simulink model "PubIfDecisionTOS_MDL"  (R2020b)
settings: configuration reference "DspaceConfig" (kept outside this file)
PostLoadFcn:
  | if any(exist('dsrtsu_mdlpostloadfcn', 'file') ~= 0), dsrtsu_mdlpostloadfcn('Execute', bdroot); end
InitFcn:
  | , if any(exist('dsmpb_private', 'file') ~= 0), dsmpb_private('dsmpb_mdlclblib', 'Init', bdroot); end,
undefined symbols (not defined in the file or in its folder): C_TOS_ACCEgoRAxletoFbumplength_m, C_TOS_ACCTargetFront_Flag, C_TOS_AEBJAPedObjDxThre_Val, C_TOS_AEBJAPedObjDyThre_Val, C_TOS_AEBJATargetSize_Val, C_TOS_AEBJAVehObjDxThre_Val, C_TOS_AEBJAVehObjDyThre_Val, C_TOS_AEBJuncPedTargetSize_Val, C_TOS_AEBLatObjDxThre_Val, C_TOS_AEBLatPedDyThre_Val, C_TOS_AEBLatTargetSize_Val, C_TOS_AEBLongTargetInEgoFront_Flag, C_TOS_axAbsGround_Parameter, C_TOS_CameraConfirmedFlag, C_TOS_CNsubjWidth, C_TOS_CurrentLaneCoreMinWidth_Val, C_TOS_CutInProb_Val_Zero, C_TOS_CutOutProb_Val_Zero, C_TOS_D2R_Val, C_TOS_DefaultValueObjectToCenterLine_dy, C_TOS_EgoCarWidth_Val, C_TOS_EgoDxRefPoint_m, C_TOS_EgoRAxletoFbumplength_m, C_TOS_HalfWidthVehicle_Con, C_TOS_HWA_CurrentLaneFlag, C_TOS_HWA_LeftLaneFlag, C_TOS_HWA_MovingDir_Vaild, C_TOS_HWA_MovState_Vaild, C_TOS_HWA_RightLaneFlag, C_TOS_LaneLineCourseErrorFront, C_TOS_LaneLineCourseErrorRear, C_TOS_MotorbikeDefaultWidth_m, C_TOS_NumberOfEffectiveTargets, C_TOS_Obj_Age_Val, C_TOS_Objdx_Constraint_Val, C_TOS_ObjectDefaultWidth_m, C_TOS_ObjInCurrentLane_Val, C_TOS_ObjInCurrentLaneValid, C_TOS_ObjInLeftLaneValid, C_TOS_ObjInRightLaneValid, C_TOS_ObjNotInCurrentLane_Val, C_TOS_ObjNotREElementType, C_TOS_ObjPredictDis_dy_ConstantVal_Zeros, C_TOS_ObjToCenterLine_ConstantVal_Zeros, C_TOS_OFMObjIDInvilad_Val, C_TOS_PIL_LatDisCons_Val_zero, C_TOS_PIL_ObjectCutInFlag_b, C_TOS_PIL_ObjectCutOutFlag_b, C_TOS_PIL_ObjLaneProb_al_Val, C_TOS_PP_ObjFusType_FC_Confirm_b, C_TOS_PP_ObjFusType_FC_FR_Confirm_b, C_TOS_PP_ObjFusType_FR_Confirm_b, C_TOS_RE_80BoolDefault_Val, C_TOS_RE_80Single181Default_Val, C_TOS_RE_80Single255Default_Val, C_TOS_RE_80Uint8Default_Val, C_TOS_RE_D2R, C_TOS_RE_D_180_Val, C_TOS_RE_InvalidObjectID_Val, C_TOS_RE_InvalidTargetChainDir_Val ... (+142)
libraries: simulink x1650, TOS_LIB x361, canfdmsglib x14
(part 59 of 69)

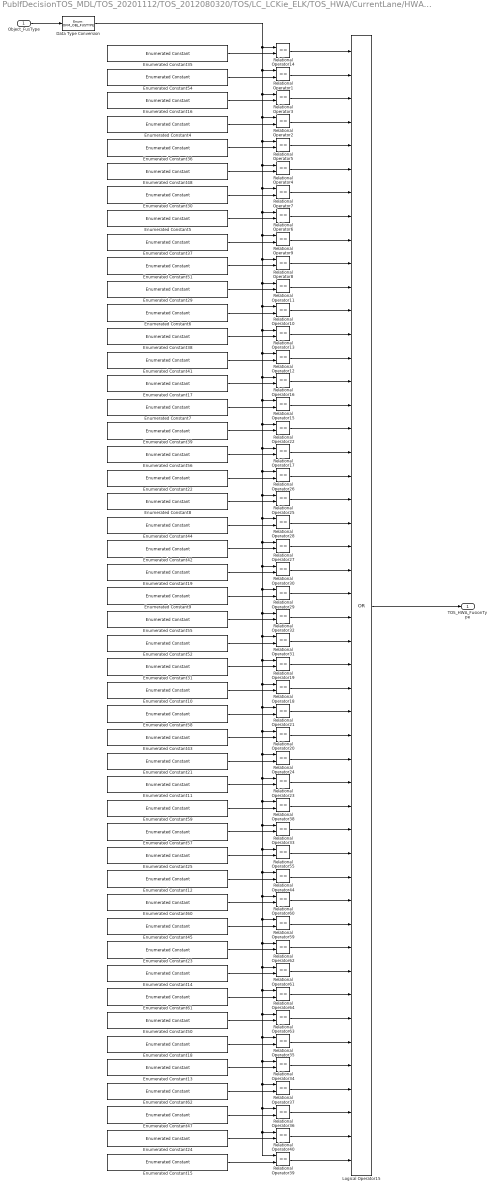
== system PubIfDecisionTOS_MDL/TOS_20201112/TOS_2012080320/TOS/LC_LCKie_ELK/TOS_HWA/CurrentLane/HWA_CurrentLane_Target/HWA_CLF_Target_3/HWA_CLR_Target/HWA_CLR_Target/HWA_CurrentRear_FusionType/FusionType ==
  Object_FusType : Inport
  Data Type Conversion : DataTypeConversion  OutDataTypeStr=Enum: OFM_OBJ_FUSTYPE
  Enumerated Constant10 : simulink/Sources/Enumerated Constant  OutDataTypeStr=Enum: OFM_OBJ_FUSTYPE  Value=OFM_OBJ_FUSTYPE.FC_FR_CR_BR  SampleTime=inf
      settings: AttributesFormatString=OFM_OBJ_FUSTYPE.FC_FR_CR_BR=43
  Enumerated Constant11 : simulink/Sources/Enumerated Constant  OutDataTypeStr=Enum: OFM_OBJ_FUSTYPE  Value=OFM_OBJ_FUSTYPE.FC_FR_CL_CR_BR  SampleTime=inf
      settings: AttributesFormatString=OFM_OBJ_FUSTYPE.FC_FR_CL_CR_BR=47
  Enumerated Constant12 : simulink/Sources/Enumerated Constant  OutDataTypeStr=Enum: OFM_OBJ_FUSTYPE  Value=OFM_OBJ_FUSTYPE.FC_FR_BL_BR  SampleTime=inf
      settings: AttributesFormatString=OFM_OBJ_FUSTYPE.FC_FR_BL_BR=51
  Enumerated Constant13 : simulink/Sources/Enumerated Constant  OutDataTypeStr=Enum: OFM_OBJ_FUSTYPE  Value=OFM_OBJ_FUSTYPE.FC_FR_CR_BL_BR  SampleTime=inf
      settings: AttributesFormatString=OFM_OBJ_FUSTYPE.FC_FR_CR_BL_BR=59
  Enumerated Constant14 : simulink/Sources/Enumerated Constant  OutDataTypeStr=Enum: OFM_OBJ_FUSTYPE  Value=OFM_OBJ_FUSTYPE.FC_FR_CL_BL_BR  SampleTime=inf
      settings: AttributesFormatString=OFM_OBJ_FUSTYPE.FC_FR_CL_BL_BR=55
  Enumerated Constant15 : simulink/Sources/Enumerated Constant  OutDataTypeStr=Enum: OFM_OBJ_FUSTYPE  Value=OFM_OBJ_FUSTYPE.FC_FR_CL_CR_BL_BR  SampleTime=inf
      settings: AttributesFormatString=OFM_OBJ_FUSTYPE.FC_FR_CL_CR_BL_BR=63
  Enumerated Constant16 : simulink/Sources/Enumerated Constant  OutDataTypeStr=Enum: OFM_OBJ_FUSTYPE  Value=OFM_OBJ_FUSTYPE.FR_BL  SampleTime=inf
      settings: AttributesFormatString=OFM_OBJ_FUSTYPE.FR_BL = 18
  Enumerated Constant17 : simulink/Sources/Enumerated Constant  OutDataTypeStr=Enum: OFM_OBJ_FUSTYPE  Value=OFM_OBJ_FUSTYPE.FR_CL_CR_BL  SampleTime=inf
      settings: AttributesFormatString=OFM_OBJ_FUSTYPE.FR_CL_CR_BL = 30
  Enumerated Constant18 : simulink/Sources/Enumerated Constant  OutDataTypeStr=Enum: OFM_OBJ_FUSTYPE  Value=OFM_OBJ_FUSTYPE.FR_CR_BL_BR  SampleTime=inf
      settings: AttributesFormatString=OFM_OBJ_FUSTYPE.FR_CR_BL_BR = 58
  Enumerated Constant19 : simulink/Sources/Enumerated Constant  OutDataTypeStr=Enum: OFM_OBJ_FUSTYPE  Value=OFM_OBJ_FUSTYPE.FR_CL_BR  SampleTime=inf
      settings: AttributesFormatString=OFM_OBJ_FUSTYPE.FR_CL_BR = 38
  Enumerated Constant21 : simulink/Sources/Enumerated Constant  OutDataTypeStr=Enum: OFM_OBJ_FUSTYPE  Value=OFM_OBJ_FUSTYPE.FR_CL_CR_BR  SampleTime=inf
      settings: AttributesFormatString=OFM_OBJ_FUSTYPE.FR_CL_CR_BR = 46
  Enumerated Constant22 : simulink/Sources/Enumerated Constant  OutDataTypeStr=Enum: OFM_OBJ_FUSTYPE  Value=OFM_OBJ_FUSTYPE.FR_BR  SampleTime=inf
      settings: AttributesFormatString=OFM_OBJ_FUSTYPE.FR_BR = 34
  Enumerated Constant23 : simulink/Sources/Enumerated Constant  OutDataTypeStr=Enum: OFM_OBJ_FUSTYPE  Value=OFM_OBJ_FUSTYPE.FR_CL_BL_BR  SampleTime=inf
      settings: AttributesFormatString=OFM_OBJ_FUSTYPE.FR_CL_BL_BR = 54
  Enumerated Constant24 : simulink/Sources/Enumerated Constant  OutDataTypeStr=Enum: OFM_OBJ_FUSTYPE  Value=OFM_OBJ_FUSTYPE.FR_CL_CR_BL_BR  SampleTime=inf
      settings: AttributesFormatString=OFM_OBJ_FUSTYPE.FR_CL_CR_BL_BR = 62
  Enumerated Constant25 : simulink/Sources/Enumerated Constant  OutDataTypeStr=Enum: OFM_OBJ_FUSTYPE  Value=OFM_OBJ_FUSTYPE.FR_BL_BR  SampleTime=inf
      settings: AttributesFormatString=OFM_OBJ_FUSTYPE.FR_BL_BR = 50
  Enumerated Constant29 : simulink/Sources/Enumerated Constant  OutDataTypeStr=Enum: OFM_OBJ_FUSTYPE  Value=OFM_OBJ_FUSTYPE.FR_CR_BL  SampleTime=inf
      settings: AttributesFormatString=OFM_OBJ_FUSTYPE.FR_CR_BL = 26
  Enumerated Constant30 : simulink/Sources/Enumerated Constant  OutDataTypeStr=Enum: OFM_OBJ_FUSTYPE  Value=OFM_OBJ_FUSTYPE.FR_CL_BL  SampleTime=inf
      settings: AttributesFormatString=OFM_OBJ_FUSTYPE.FR_CL_BL = 22
  Enumerated Constant31 : simulink/Sources/Enumerated Constant  OutDataTypeStr=Enum: OFM_OBJ_FUSTYPE  Value=OFM_OBJ_FUSTYPE.FR_CR_BR  SampleTime=inf
      settings: AttributesFormatString=OFM_OBJ_FUSTYPE.FR_CR_BR = 42
  Enumerated Constant35 : simulink/Sources/Enumerated Constant  OutDataTypeStr=Enum: OFM_OBJ_FUSTYPE  Value=OFM_OBJ_FUSTYPE.BL  SampleTime=inf
      settings: AttributesFormatString=OFM_OBJ_FUSTYPE.BL = 16
  Enumerated Constant36 : simulink/Sources/Enumerated Constant  OutDataTypeStr=Enum: OFM_OBJ_FUSTYPE  Value=OFM_OBJ_FUSTYPE.CL_BL  SampleTime=inf
      settings: AttributesFormatString=OFM_OBJ_FUSTYPE.CL_BL=20
  Enumerated Constant37 : simulink/Sources/Enumerated Constant  OutDataTypeStr=Enum: OFM_OBJ_FUSTYPE  Value=OFM_OBJ_FUSTYPE.CR_BL  SampleTime=inf
      settings: AttributesFormatString=OFM_OBJ_FUSTYPE.CR_BL = 24
  Enumerated Constant38 : simulink/Sources/Enumerated Constant  OutDataTypeStr=Enum: OFM_OBJ_FUSTYPE  Value=OFM_OBJ_FUSTYPE.CL_CR_BL  SampleTime=inf
      settings: AttributesFormatString=OFM_OBJ_FUSTYPE.CL_CR_BL=28
  Enumerated Constant39 : simulink/Sources/Enumerated Constant  OutDataTypeStr=Enum: OFM_OBJ_FUSTYPE  Value=OFM_OBJ_FUSTYPE.BR  SampleTime=inf
      settings: AttributesFormatString=OFM_OBJ_FUSTYPE.BR = 32
  Enumerated Constant4 : simulink/Sources/Enumerated Constant  OutDataTypeStr=Enum: OFM_OBJ_FUSTYPE  Value=OFM_OBJ_FUSTYPE.FC_FR_BL  SampleTime=inf
      settings: AttributesFormatString=OFM_OBJ_FUSTYPE.FC_FR_BL=19
  Enumerated Constant41 : simulink/Sources/Enumerated Constant  OutDataTypeStr=Enum: OFM_OBJ_FUSTYPE  Value=OFM_OBJ_FUSTYPE.FC_CL_CR_BL  SampleTime=inf
      settings: AttributesFormatString=OFM_OBJ_FUSTYPE.FC_CL_CR_BL = 29
  Enumerated Constant42 : simulink/Sources/Enumerated Constant  OutDataTypeStr=Enum: OFM_OBJ_FUSTYPE  Value=OFM_OBJ_FUSTYPE.FC_CL_BR  SampleTime=inf
      settings: AttributesFormatString=OFM_OBJ_FUSTYPE.FC_CL_BR = 37
  Enumerated Constant43 : simulink/Sources/Enumerated Constant  OutDataTypeStr=Enum: OFM_OBJ_FUSTYPE  Value=OFM_OBJ_FUSTYPE.FC_CL_CR_BR  SampleTime=inf
      settings: AttributesFormatString=OFM_OBJ_FUSTYPE.FC_CL_CR_BR = 45
  Enumerated Constant44 : simulink/Sources/Enumerated Constant  OutDataTypeStr=Enum: OFM_OBJ_FUSTYPE  Value=OFM_OBJ_FUSTYPE.CL_BR  SampleTime=inf
      settings: AttributesFormatString=OFM_OBJ_FUSTYPE.CL_BR = 36
  Enumerated Constant45 : simulink/Sources/Enumerated Constant  OutDataTypeStr=Enum: OFM_OBJ_FUSTYPE  Value=OFM_OBJ_FUSTYPE.FC_CL_BL_BR  SampleTime=inf
      settings: AttributesFormatString=OFM_OBJ_FUSTYPE.FC_CL_BL_BR = 53
  Enumerated Constant47 : simulink/Sources/Enumerated Constant  OutDataTypeStr=Enum: OFM_OBJ_FUSTYPE  Value=OFM_OBJ_FUSTYPE.FC_CL_CR_BL_BR  SampleTime=inf
      settings: AttributesFormatString=OFM_OBJ_FUSTYPE.FC_CL_CR_BL_BR = 61
  Enumerated Constant48 : simulink/Sources/Enumerated Constant  OutDataTypeStr=Enum: OFM_OBJ_FUSTYPE  Value=OFM_OBJ_FUSTYPE.FC_CL_BL  SampleTime=inf
      settings: AttributesFormatString=OFM_OBJ_FUSTYPE.FC_CL_BL = 21
  Enumerated Constant5 : simulink/Sources/Enumerated Constant  OutDataTypeStr=Enum: OFM_OBJ_FUSTYPE  Value=OFM_OBJ_FUSTYPE.FC_FR_CL_BL  SampleTime=inf
      settings: AttributesFormatString=OFM_OBJ_FUSTYPE.FC_FR_CL_BL=23
  Enumerated Constant50 : simulink/Sources/Enumerated Constant  OutDataTypeStr=Enum: OFM_OBJ_FUSTYPE  Value=OFM_OBJ_FUSTYPE.FC_CR_BL_BR  SampleTime=inf
      settings: AttributesFormatString=OFM_OBJ_FUSTYPE.FC_CR_BL_BR = 57
  Enumerated Constant51 : simulink/Sources/Enumerated Constant  OutDataTypeStr=Enum: OFM_OBJ_FUSTYPE  Value=OFM_OBJ_FUSTYPE.FC_CR_BL  SampleTime=inf
      settings: AttributesFormatString=OFM_OBJ_FUSTYPE.FC_CR_BL = 25
  Enumerated Constant52 : simulink/Sources/Enumerated Constant  OutDataTypeStr=Enum: OFM_OBJ_FUSTYPE  Value=OFM_OBJ_FUSTYPE.FC_CR_BR  SampleTime=inf
      settings: AttributesFormatString=OFM_OBJ_FUSTYPE.FC_CR_BR = 41
  Enumerated Constant54 : simulink/Sources/Enumerated Constant  OutDataTypeStr=Enum: OFM_OBJ_FUSTYPE  Value=OFM_OBJ_FUSTYPE.FC_BL  SampleTime=inf
      settings: AttributesFormatString=OFM_OBJ_FUSTYPE.FC_BL = 17
  Enumerated Constant55 : simulink/Sources/Enumerated Constant  OutDataTypeStr=Enum: OFM_OBJ_FUSTYPE  Value=OFM_OBJ_FUSTYPE.CR_BR  SampleTime=inf
      settings: AttributesFormatString=OFM_OBJ_FUSTYPE.CR_BR = 40
  Enumerated Constant56 : simulink/Sources/Enumerated Constant  OutDataTypeStr=Enum: OFM_OBJ_FUSTYPE  Value=OFM_OBJ_FUSTYPE.FC_BR  SampleTime=inf
      settings: AttributesFormatString=OFM_OBJ_FUSTYPE.FC_BR = 33
  Enumerated Constant57 : simulink/Sources/Enumerated Constant  OutDataTypeStr=Enum: OFM_OBJ_FUSTYPE  Value=OFM_OBJ_FUSTYPE.FC_BL_BR  SampleTime=inf
      settings: AttributesFormatString=OFM_OBJ_FUSTYPE.FC_BL_BR = 49
  Enumerated Constant58 : simulink/Sources/Enumerated Constant  OutDataTypeStr=Enum: OFM_OBJ_FUSTYPE  Value=OFM_OBJ_FUSTYPE.CL_CR_BR  SampleTime=inf
      settings: AttributesFormatString=OFM_OBJ_FUSTYPE.CL_CR_BR = 44
  Enumerated Constant59 : simulink/Sources/Enumerated Constant  OutDataTypeStr=Enum: OFM_OBJ_FUSTYPE  Value=OFM_OBJ_FUSTYPE.BL_BR  SampleTime=inf
      settings: AttributesFormatString=OFM_OBJ_FUSTYPE.BL_BR = 48
  Enumerated Constant6 : simulink/Sources/Enumerated Constant  OutDataTypeStr=Enum: OFM_OBJ_FUSTYPE  Value=OFM_OBJ_FUSTYPE.FC_FR_CR_BL  SampleTime=inf
      settings: AttributesFormatString=OFM_OBJ_FUSTYPE.FC_FR_CR_BL=27
  Enumerated Constant60 : simulink/Sources/Enumerated Constant  OutDataTypeStr=Enum: OFM_OBJ_FUSTYPE  Value=OFM_OBJ_FUSTYPE.CL_BL_BR  SampleTime=inf
      settings: AttributesFormatString=OFM_OBJ_FUSTYPE.CL_BL_BR = 52
  Enumerated Constant61 : simulink/Sources/Enumerated Constant  OutDataTypeStr=Enum: OFM_OBJ_FUSTYPE  Value=OFM_OBJ_FUSTYPE.CR_BL_BR  SampleTime=inf
      settings: AttributesFormatString=OFM_OBJ_FUSTYPE.CR_BL_BR = 56
  Enumerated Constant62 : simulink/Sources/Enumerated Constant  OutDataTypeStr=Enum: OFM_OBJ_FUSTYPE  Value=OFM_OBJ_FUSTYPE.CL_CR_BL_BR  SampleTime=inf
      settings: AttributesFormatString=OFM_OBJ_FUSTYPE.CL_CR_BL_BR = 60
  Enumerated Constant7 : simulink/Sources/Enumerated Constant  OutDataTypeStr=Enum: OFM_OBJ_FUSTYPE  Value=OFM_OBJ_FUSTYPE.FC_FR_CL_CR_BL  SampleTime=inf
      settings: AttributesFormatString=OFM_OBJ_FUSTYPE.FC_FR_CL_CR_BL=31
  Enumerated Constant8 : simulink/Sources/Enumerated Constant  OutDataTypeStr=Enum: OFM_OBJ_FUSTYPE  Value=OFM_OBJ_FUSTYPE.FC_FR_BR  SampleTime=inf
      settings: AttributesFormatString=OFM_OBJ_FUSTYPE.FC_FR_BR=35
  Enumerated Constant9 : simulink/Sources/Enumerated Constant  OutDataTypeStr=Enum: OFM_OBJ_FUSTYPE  Value=OFM_OBJ_FUSTYPE.FC_FR_CL_BR  SampleTime=inf
      settings: AttributesFormatString=OFM_OBJ_FUSTYPE.FC_FR_CL_BR=39
  Logical Operator15 : Logic  Operator=OR  Inputs=48  AllPortsSameDT=off  OutDataTypeStr=boolean
  Relational Operator{1..40,44,55,59..64} (48 alike) : RelationalOperator  Operator===  OutDataTypeStr=boolean  RndMeth=Nearest
  TOS_HWA_FusionType : Outport
  wires:
  Relational Operator12/1 -> Logical Operator15/14
  Data Type Conversion/1 -> Relational Operator14/1, Relational Operator35/1, Relational Operator39/1, Relational Operator40/1, Relational Operator36/1, Relational Operator37/1, Relational Operator34/1, Relational Operator63/1, Relational Operator64/1, Relational Operator61/1, Relational Operator62/1, Relational Operator59/1, Relational Operator60/1, Relational Operator44/1, Relational Operator55/1, Relational Operator33/1, Relational Operator38/1, Relational Operator23/1, Relational Operator24/1, Relational Operator20/1, Relational Operator21/1, Relational Operator18/1, Relational Operator19/1, Relational Operator31/1, Relational Operator32/1, Relational Operator29/1, Relational Operator30/1, Relational Operator27/1, Relational Operator28/1, Relational Operator25/1, Relational Operator26/1, Relational Operator17/1, Relational Operator22/1, Relational Operator15/1, Relational Operator16/1, Relational Operator12/1, Relational Operator13/1, Relational Operator10/1, Relational Operator11/1, Relational Operator8/1, Relational Operator9/1, Relational Operator6/1, Relational Operator7/1, Relational Operator4/1, Relational Operator5/1, Relational Operator2/1, Relational Operator3/1, Relational Operator1/1
  Enumerated Constant39/1 -> Relational Operator22/2
  Relational Operator14/1 -> Logical Operator15/1
  Enumerated Constant36/1 -> Relational Operator5/2
  Relational Operator55/1 -> Logical Operator15/35
  Relational Operator31/1 -> Logical Operator15/26
  Enumerated Constant62/1 -> Relational Operator37/2
  Enumerated Constant42/1 -> Relational Operator27/2
  Relational Operator62/1 -> Logical Operator15/39
  Enumerated Constant17/1 -> Relational Operator16/2
  Relational Operator30/1 -> Logical Operator15/23
  Enumerated Constant10/1 -> Relational Operator18/2
  Enumerated Constant52/1 -> Relational Operator31/2
  Enumerated Constant56/1 -> Relational Operator17/2
  Enumerated Constant29/1 -> Relational Operator11/2
  Enumerated Constant51/1 -> Relational Operator8/2
  Enumerated Constant24/1 -> Relational Operator40/2
  Relational Operator39/1 -> Logical Operator15/48
  Relational Operator32/1 -> Logical Operator15/25
  Relational Operator5/1 -> Logical Operator15/5
  Object_FusType/1 -> Data Type Conversion/1
  Relational Operator37/1 -> Logical Operator15/45
  Enumerated Constant38/1 -> Relational Operator13/2
  Enumerated Constant13/1 -> Relational Operator34/2
  Enumerated Constant47/1 -> Relational Operator36/2
  Enumerated Constant8/1 -> Relational Operator25/2
  Relational Operator4/1 -> Logical Operator15/6
  Relational Operator2/1 -> Logical Operator15/4
  Relational Operator40/1 -> Logical Operator15/47
  Enumerated Constant61/1 -> Relational Operator64/2
  Enumerated Constant60/1 -> Relational Operator60/2
  Relational Operator21/1 -> Logical Operator15/29
  Relational Operator24/1 -> Logical Operator15/31
  Enumerated Constant25/1 -> Relational Operator55/2
  Relational Operator10/1 -> Logical Operator15/12
  Enumerated Constant5/1 -> Relational Operator6/2
  Enumerated Constant18/1 -> Relational Operator35/2
  Relational Operator19/1 -> Logical Operator15/27
  Relational Operator61/1 -> Logical Operator15/40
  Enumerated Constant43/1 -> Relational Operator20/2
  Enumerated Constant55/1 -> Relational Operator32/2
  Enumerated Constant31/1 -> Relational Operator19/2
  Relational Operator20/1 -> Logical Operator15/30
  Relational Operator36/1 -> Logical Operator15/46
  Enumerated Constant14/1 -> Relational Operator61/2
  Enumerated Constant11/1 -> Relational Operator23/2
  Enumerated Constant12/1 -> Relational Operator44/2
  Relational Operator18/1 -> Logical Operator15/28
  Enumerated Constant45/1 -> Relational Operator59/2
  Relational Operator60/1 -> Logical Operator15/37
  Relational Operator26/1 -> Logical Operator15/19
  Relational Operator11/1 -> Logical Operator15/11
  Enumerated Constant9/1 -> Relational Operator29/2
  Relational Operator6/1 -> Logical Operator15/8
  Enumerated Constant21/1 -> Relational Operator24/2
  Enumerated Constant59/1 -> Relational Operator38/2
  Enumerated Constant37/1 -> Relational Operator9/2
  Enumerated Constant35/1 -> Relational Operator14/2
  Relational Operator22/1 -> Logical Operator15/17
  Enumerated Constant22/1 -> Relational Operator26/2
  Relational Operator59/1 -> Logical Operator15/38
  Relational Operator15/1 -> Logical Operator15/16
  Relational Operator34/1 -> Logical Operator15/44
  Relational Operator44/1 -> Logical Operator15/36
  Enumerated Constant6/1 -> Relational Operator10/2
  Relational Operator63/1 -> Logical Operator15/42
  Relational Operator35/1 -> Logical Operator15/43
  Relational Operator64/1 -> Logical Operator15/41
  Enumerated Constant7/1 -> Relational Operator15/2
  Enumerated Constant41/1 -> Relational Operator12/2
  Relational Operator1/1 -> Logical Operator15/2
  Relational Operator25/1 -> Logical Operator15/20
  Relational Operator17/1 -> Logical Operator15/18
  Enumerated Constant30/1 -> Relational Operator7/2
  Enumerated Constant19/1 -> Relational Operator30/2
  Relational Operator33/1 -> Logical Operator15/34
  Enumerated Constant57/1 -> Relational Operator33/2
  Relational Operator9/1 -> Logical Operator15/9
  Enumerated Constant4/1 -> Relational Operator2/2
  Enumerated Constant16/1 -> Relational Operator3/2
  Relational Operator38/1 -> Logical Operator15/33
  Relational Operator3/1 -> Logical Operator15/3
  Relational Operator13/1 -> Logical Operator15/13
  Relational Operator23/1 -> Logical Operator15/32
  Logical Operator15/1 -> TOS_HWA_FusionType/1
  Relational Operator28/1 -> Logical Operator15/21
  Enumerated Constant23/1 -> Relational Operator62/2
  Enumerated Constant48/1 -> Relational Operator4/2
  Enumerated Constant44/1 -> Relational Operator28/2
  Relational Operator16/1 -> Logical Operator15/15
  Enumerated Constant58/1 -> Relational Operator21/2
  Enumerated Constant54/1 -> Relational Operator1/2
  Relational Operator7/1 -> Logical Operator15/7
  Relational Operator27/1 -> Logical Operator15/22
  Relational Operator8/1 -> Logical Operator15/10
  Enumerated Constant15/1 -> Relational Operator39/2
  Enumerated Constant50/1 -> Relational Operator63/2
  Relational Operator29/1 -> Logical Operator15/24

== system PubIfDecisionTOS_MDL/TOS_20201112/TOS_2012080320/TOS/LC_LCKie_ELK/TOS_HWA/LeftLane/TOS_HWA_LeftLane/TOS_HWA_LeftLane/TOS_HWA/HWA_LeftLane/HWA_LeftLane_Front/HWA_InLeftLane_Flag ==
  HWA_InRightLane : Inport
  Compare To Constant3 : simulink/Logic and Bit Operations/Compare To Constant  relop===  const=C_TOS_HWA_RightLaneFlag  OutDataTypeStr=boolean
      settings: AttributesFormatString=C_TOS_HWA_RightLaneFlag = 1
  TOS_HWA_InLeftLane_Flag : Outport
  wires:
  Compare To Constant3/1 -> TOS_HWA_InLeftLane_Flag/1
  HWA_InRightLane/1 -> Compare To Constant3/1

== system PubIfDecisionTOS_MDL/TOS_20201112/TOS_2012080320/TOS/LC_LCKie_ELK/TOS_HWA/LeftLane/TOS_HWA_LeftLane/TOS_HWA_LeftLane/TOS_HWA/HWA_LeftLane/HWA_LeftLane_Front/HWA_LeftFront_FusType ==
  object_MovingState : Inport
  PP_ObjFusType_FR_Confirm : Inport  Port=2
  PP_ObjFusType_FC_Confirm : Inport  Port=3
  HWA_MovState_InternalSig : Inport  Port=4
  Object_DX : Inport  Port=5
  Compare To Constant1 : simulink/Logic and Bit Operations/Compare To Constant  relop===  const=C_TOS_HWA_MovState_Vaild  OutDataTypeStr=boolean
      settings: AttributesFormatString=C_TOS_HWA_MovState_Vaild = 1
  Compare To Constant10 : simulink/Logic and Bit Operations/Compare To Constant  relop===  const=OFM_OBJ_MOVINGSTATE_E.STOPPED  OutDataTypeStr=boolean
      settings: AttributesFormatString=OFM_OBJ_MOVINGSTATE_E.STOPPED = 4
  Compare To Constant11 : simulink/Logic and Bit Operations/Compare To Constant  relop===  const=C_TOS_PP_ObjFusType_FC_Confirm_b  OutDataTypeStr=boolean
      settings: AttributesFormatString=C_TOS_PP_ObjFusType_FC_Confirm_b = 1
  Compare To Constant12 : simulink/Logic and Bit Operations/Compare To Constant  relop===  const=C_TOS_PP_ObjFusType_FR_Confirm_b  OutDataTypeStr=boolean
      settings: AttributesFormatString=C_TOS_PP_ObjFusType_FR_Confirm_b = 1
  Compare To Constant13 : simulink/Logic and Bit Operations/Compare To Constant  relop===  const=C_TOS_PP_ObjFusType_FC_Confirm_b  OutDataTypeStr=boolean
      settings: AttributesFormatString=C_TOS_PP_ObjFusType_FC_Confirm_b = 1
  Compare To Constant2 : simulink/Logic and Bit Operations/Compare To Constant  relop=>  const=P_TOS_RefPoint_FixDis_dx2_m  OutDataTypeStr=boolean
      settings: AttributesFormatString=P_TOS_RefPoint_FixDis_dx2_m = 3 m
  Compare To Constant3 : simulink/Logic and Bit Operations/Compare To Constant  relop===  const=C_TOS_HWA_MovState_Vaild  OutDataTypeStr=boolean
      settings: AttributesFormatString=C_TOS_HWA_MovState_Vaild = 1
  Compare To Constant6 : simulink/Logic and Bit Operations/Compare To Constant  relop===  const=OFM_OBJ_MOVINGSTATE_E.MOVING  OutDataTypeStr=boolean
      settings: AttributesFormatString=OFM_OBJ_MOVINGSTATE_E.MOVING = 2
  Compare To Constant7 : simulink/Logic and Bit Operations/Compare To Constant  relop===  const=OFM_OBJ_MOVINGSTATE_E.MOVING_SLOWLY  OutDataTypeStr=boolean
      settings: AttributesFormatString=OFM_OBJ_MOVINGSTATE_E.MOVING_SLOWLY = 5
  Compare To Constant8 : simulink/Logic and Bit Operations/Compare To Constant  relop===  const=OFM_OBJ_MOVINGSTATE_E.UNKNOWN  OutDataTypeStr=boolean
      settings: AttributesFormatString=OFM_OBJ_MOVINGSTATE_E.UNKNOWN = 1
  Compare To Constant9 : simulink/Logic and Bit Operations/Compare To Constant  relop===  const=OFM_OBJ_MOVINGSTATE_E.STATIONARY  OutDataTypeStr=boolean
      settings: AttributesFormatString=OFM_OBJ_MOVINGSTATE_E.STATIONARY = 3
  Constant : Constant  OutDataTypeStr=boolean
  Data Type Conversion1 : DataTypeConversion  OutDataTypeStr=Enum: OFM_OBJ_MOVINGSTATE_E
  Logical Operator15 : Logic  AllPortsSameDT=off  OutDataTypeStr=boolean
  Logical Operator3 : Logic  AllPortsSameDT=off  OutDataTypeStr=boolean
  Logical Operator5 : Logic  Operator=OR  Inputs=4  AllPortsSameDT=off  OutDataTypeStr=boolean
  Logical Operator6 : Logic  Operator=OR  AllPortsSameDT=off  OutDataTypeStr=boolean
  Logical Operator7 : Logic  Operator=OR  Inputs=3  AllPortsSameDT=off  OutDataTypeStr=boolean
  Logical Operator8 : Logic  Operator=OR  AllPortsSameDT=off  OutDataTypeStr=boolean
  Switch : Switch  Criteria=u2 > Threshold
  TOS_HWA_LeftFront_FusType : Outport
  wires:
  Constant/1 -> Switch/3
  Compare To Constant2/1 -> Switch/2
  Logical Operator6/1 -> Switch/1
  Object_DX/1 -> Compare To Constant2/1
  Compare To Constant1/1 -> Logical Operator7/3
  Compare To Constant3/1 -> Logical Operator5/4
  HWA_MovState_InternalSig/1 -> Compare To Constant3/1, Compare To Constant1/1
  Logical Operator3/1 -> Logical Operator6/2
  object_MovingState/1 -> Data Type Conversion1/1
  Logical Operator8/1 -> Logical Operator15/1
  Compare To Constant7/1 -> Logical Operator5/2
  Compare To Constant13/1 -> Logical Operator3/1
  Compare To Constant9/1 -> Logical Operator7/1
  Logical Operator7/1 -> Logical Operator3/2
  Logical Operator15/1 -> Logical Operator6/1
  Data Type Conversion1/1 -> Compare To Constant7/1, Compare To Constant10/1, Compare To Constant8/1, Compare To Constant9/1, Compare To Constant6/1
  Compare To Constant10/1 -> Logical Operator5/3
  Compare To Constant11/1 -> Logical Operator8/2
  Compare To Constant12/1 -> Logical Operator8/1
  Compare To Constant8/1 -> Logical Operator7/2
  PP_ObjFusType_FC_Confirm/1 -> Compare To Constant11/1, Compare To Constant13/1
  Compare To Constant6/1 -> Logical Operator5/1
  Logical Operator5/1 -> Logical Operator15/2
  PP_ObjFusType_FR_Confirm/1 -> Compare To Constant12/1
  Switch/1 -> TOS_HWA_LeftFront_FusType/1

== system PubIfDecisionTOS_MDL/TOS_20201112/TOS_2012080320/TOS/LC_LCKie_ELK/TOS_HWA/LeftLane/TOS_HWA_LeftLane/TOS_HWA_LeftLane/TOS_HWA/HWA_LeftLane/HWA_LeftLane_Front/HWA_LeftFront_TargMovDir ==
  HWA_MovingDir_InternalSig : Inport
  Compare To Constant3 : simulink/Logic and Bit Operations/Compare To Constant  relop===  const=C_TOS_HWA_MovingDir_Vaild  OutDataTypeStr=boolean
      settings: AttributesFormatString=C_TOS_HWA_MovingDir_Vaild = 1
  TOS_HWA_LeftFront_TargMovDir : Outport
  wires:
  Compare To Constant3/1 -> TOS_HWA_LeftFront_TargMovDir/1
  HWA_MovingDir_InternalSig/1 -> Compare To Constant3/1

== system PubIfDecisionTOS_MDL/TOS_20201112/TOS_2012080320/TOS/LC_LCKie_ELK/TOS_HWA/LeftLane/TOS_HWA_LeftLane/TOS_HWA_LeftLane/TOS_HWA/HWA_LeftLane/HWA_LeftLane_Front/HWA_LeftRear_Default ==
  Constant{,2..6} (6 alike) : Constant  Value=0  OutDataTypeStr=boolean
  TOS_HWA_LeftRear_TargConfirm_b : Outport
  TOS_HWA_LeftRear_MovState_ObserVale : Outport  Port=2
  TOS_HWA_LeftRear_FusionType_ObserVale : Outport  Port=3
  TOS_HWA_InLeftLane_Rear_Flag_ObserVale : Outport  Port=4
  TOS_HWA_LeftRear_TargetMovingDir_ObserVale : Outport  Port=5
  TOS_HWA_LeftRear_DyConfirm_ObserVale : Outport  Port=6
  wires:
  Constant4/1 -> TOS_HWA_InLeftLane_Rear_Flag_ObserVale/1
  Constant5/1 -> TOS_HWA_LeftRear_TargetMovingDir_ObserVale/1
  Constant6/1 -> TOS_HWA_LeftRear_DyConfirm_ObserVale/1
  Constant2/1 -> TOS_HWA_LeftRear_MovState_ObserVale/1
  Constant3/1 -> TOS_HWA_LeftRear_FusionType_ObserVale/1
  Constant/1 -> TOS_HWA_LeftRear_TargConfirm_b/1

== system PubIfDecisionTOS_MDL/TOS_20201112/TOS_2012080320/TOS/LC_LCKie_ELK/TOS_HWA/LeftLane/TOS_HWA_LeftLane/TOS_HWA_LeftLane/TOS_HWA/HWA_LeftLane/HWA_LeftLane_Rear/HWA_InLeftLane_Flag ==
  HWA_InRightLane : Inport
  Compare To Constant1 : simulink/Logic and Bit Operations/Compare To Constant  relop===  const=C_TOS_HWA_LeftLaneFlag  OutDataTypeStr=boolean
      settings: AttributesFormatString=C_TOS_HWA_LeftLaneFlag = 1
  TOS_HWA_InLeftLane_Flag : Outport
  wires:
  Compare To Constant1/1 -> TOS_HWA_InLeftLane_Flag/1
  HWA_InRightLane/1 -> Compare To Constant1/1

== system PubIfDecisionTOS_MDL/TOS_20201112/TOS_2012080320/TOS/LC_LCKie_ELK/TOS_HWA/LeftLane/TOS_HWA_LeftLane/TOS_HWA_LeftLane/TOS_HWA/HWA_LeftLane/HWA_LeftLane_Rear/HWA_LeftFront_Default ==
  Constant{1,7..9} (4 alike) : Constant  Value=0  OutDataTypeStr=boolean
  TOS_HWA_LeftFront_TargConfirm_b : Outport
  TOS_HWA_LeftFront_FusType_ObserVale : Outport  Port=2
  TOS_HWA_InLeftLane_Front_Flag_ObserVale : Outport  Port=3
  TOS_HWA_LeftFront_TargMovDir_ObserVale : Outport  Port=4
  wires:
  Constant1/1 -> TOS_HWA_LeftFront_TargConfirm_b/1
  Constant7/1 -> TOS_HWA_LeftFront_FusType_ObserVale/1
  Constant9/1 -> TOS_HWA_LeftFront_TargMovDir_ObserVale/1
  Constant8/1 -> TOS_HWA_InLeftLane_Front_Flag_ObserVale/1

== system PubIfDecisionTOS_MDL/TOS_20201112/TOS_2012080320/TOS/LC_LCKie_ELK/TOS_HWA/LeftLane/TOS_HWA_LeftLane/TOS_HWA_LeftLane/TOS_HWA/HWA_LeftLane/HWA_LeftLane_Rear/HWA_LeftRear_DyConfirm ==
  Object_DY : Inport
  Object_DX : Inport  Port=2
  Abs1 : Abs
  Abs2 : Abs
  Relational Operator1 : RelationalOperator  Operator=<=  OutDataTypeStr=boolean  RndMeth=Simplest
  data3 : Lookup_n-D  NumberOfTableDimensions=1  BreakpointsForDimension1=[0,20,40,60,80,100,120]  Table=[5.75,5.75,5.75,5.75,5.75,5.75,5.75]  RndMeth=Simplest  InputSameDT=on
  TOS_HWA_LeftRear_DyConfirm : Outport
  wires:
  Relational Operator1/1 -> TOS_HWA_LeftRear_DyConfirm/1
  Abs1/1 -> Relational Operator1/1
  Object_DY/1 -> Abs1/1
  data3/1 -> Relational Operator1/2
  Abs2/1 -> data3/1
  Object_DX/1 -> Abs2/1

== system PubIfDecisionTOS_MDL/TOS_20201112/TOS_2012080320/TOS/LC_LCKie_ELK/TOS_HWA/LeftLane/TOS_HWA_LeftLane/TOS_HWA_LeftLane/TOS_HWA/HWA_LeftLane/HWA_LeftLane_Rear/HWA_LeftRear_FusionType ==
  Object_FusType : Inport
  Object_DX : Inport  Port=2
  Compare To Constant2 : simulink/Logic and Bit Operations/Compare To Constant  relop=<  const=P_TOS_RefPoint_FixDis_dx1_m  OutDataTypeStr=boolean
      settings: AttributesFormatString=P_TOS_RefPoint_FixDis_dx1_m= -3 m
  Constant : Constant  OutDataTypeStr=boolean
  FusionType : Subsystem
  Switch : Switch  Criteria=u2 > Threshold
  TOS_HWA_LeftRear_FusionType : Outport
  wires:
  Constant/1 -> Switch/3
  FusionType/1(TOS_HWA_FusionType) -> Switch/1
  Compare To Constant2/1 -> Switch/2
  Object_DX/1 -> Compare To Constant2/1
  Object_FusType/1 -> FusionType/1(Object_FusType)
  Switch/1 -> TOS_HWA_LeftRear_FusionType/1

== system PubIfDecisionTOS_MDL/TOS_20201112/TOS_2012080320/TOS/LC_LCKie_ELK/TOS_HWA/LeftLane/TOS_HWA_LeftLane/TOS_HWA_LeftLane/TOS_HWA/HWA_LeftLane/HWA_LeftLane_Rear/HWA_LeftRear_MovState ==
  HWA_MovState_InternalSig : Inport
  Compare To Constant3 : simulink/Logic and Bit Operations/Compare To Constant  relop===  const=C_TOS_HWA_MovState_Vaild  OutDataTypeStr=boolean
      settings: AttributesFormatString=C_TOS_HWA_MovState_Vaild = 1
  TOS_HWA_LeftRear_MovState : Outport
  wires:
  Compare To Constant3/1 -> TOS_HWA_LeftRear_MovState/1
  HWA_MovState_InternalSig/1 -> Compare To Constant3/1

== system PubIfDecisionTOS_MDL/TOS_20201112/TOS_2012080320/TOS/LC_LCKie_ELK/TOS_HWA/LeftLane/TOS_HWA_LeftLane/TOS_HWA_LeftLane/TOS_HWA/HWA_LeftLane/HWA_LeftLane_Rear/HWA_LeftRear_TargetMovingDir ==
  HWA_MovingDir_InternalSig : Inport
  Compare To Constant3 : simulink/Logic and Bit Operations/Compare To Constant  relop===  const=C_TOS_HWA_MovingDir_Vaild  OutDataTypeStr=boolean
      settings: AttributesFormatString=C_TOS_HWA_MovingDir_Vaild = 1
  TOS_HWA_LeftRear_TargetMovingDir : Outport
  wires:
  Compare To Constant3/1 -> TOS_HWA_LeftRear_TargetMovingDir/1
  HWA_MovingDir_InternalSig/1 -> Compare To Constant3/1

== system PubIfDecisionTOS_MDL/TOS_20201112/TOS_2012080320/TOS/LC_LCKie_ELK/TOS_HWA/RightLane/TOS_HWA_RightLane/TOS_HWA_RightLane/TOS_HWA/HWA_RightLane/HWA_RightLane_Front/HWA_InRightLane_Flag ==
  TOS_TLJ_RightLaneConfirm_Flag : Inport
  Compare To Constant3 : simulink/Logic and Bit Operations/Compare To Constant  relop===  const=C_TOS_HWA_RightLaneFlag  OutDataTypeStr=boolean
      settings: AttributesFormatString=C_TOS_HWA_RightLaneFlag = 1
  TOS_HWA_InRightLane_Flag : Outport
  wires:
  TOS_TLJ_RightLaneConfirm_Flag/1 -> Compare To Constant3/1
  Compare To Constant3/1 -> TOS_HWA_InRightLane_Flag/1

== system PubIfDecisionTOS_MDL/TOS_20201112/TOS_2012080320/TOS/LC_LCKie_ELK/TOS_HWA/RightLane/TOS_HWA_RightLane/TOS_HWA_RightLane/TOS_HWA/HWA_RightLane/HWA_RightLane_Front/HWA_RightFront_FusType ==
  object_MovingState : Inport
  PP_ObjFusType_FR_Confirm : Inport  Port=2
  PP_ObjFusType_FC_Confirm : Inport  Port=3
  HWA_MovState_InternalSig : Inport  Port=4
  Object_DX : Inport  Port=5
  Compare To Constant1 : simulink/Logic and Bit Operations/Compare To Constant  relop===  const=C_TOS_HWA_MovState_Vaild  OutDataTypeStr=boolean
      settings: AttributesFormatString=C_TOS_HWA_MovState_Vaild = 1
  Compare To Constant10 : simulink/Logic and Bit Operations/Compare To Constant  relop===  const=OFM_OBJ_MOVINGSTATE_E.STOPPED  OutDataTypeStr=boolean
      settings: AttributesFormatString=OFM_OBJ_MOVINGSTATE_E.STOPPED = 4
  Compare To Constant11 : simulink/Logic and Bit Operations/Compare To Constant  relop===  const=C_TOS_PP_ObjFusType_FC_Confirm_b  OutDataTypeStr=boolean
      settings: AttributesFormatString=C_TOS_PP_ObjFusType_FC_Confirm_b = 1
  Compare To Constant12 : simulink/Logic and Bit Operations/Compare To Constant  relop===  const=C_TOS_PP_ObjFusType_FR_Confirm_b  OutDataTypeStr=boolean
      settings: AttributesFormatString=C_TOS_PP_ObjFusType_FR_Confirm_b = 1
  Compare To Constant13 : simulink/Logic and Bit Operations/Compare To Constant  relop===  const=C_TOS_PP_ObjFusType_FC_Confirm_b  OutDataTypeStr=boolean
      settings: AttributesFormatString=C_TOS_PP_ObjFusType_FC_Confirm_b = 1
  Compare To Constant2 : simulink/Logic and Bit Operations/Compare To Constant  relop=>  const=P_TOS_RefPoint_FixDis_dx2_m  OutDataTypeStr=boolean
      settings: AttributesFormatString=P_TOS_RefPoint_FixDis_dx2_m = 3 m
  Compare To Constant3 : simulink/Logic and Bit Operations/Compare To Constant  relop===  const=C_TOS_HWA_MovState_Vaild  OutDataTypeStr=boolean
      settings: AttributesFormatString=C_TOS_HWA_MovState_Vaild = 1
  Compare To Constant6 : simulink/Logic and Bit Operations/Compare To Constant  relop===  const=OFM_OBJ_MOVINGSTATE_E.MOVING  OutDataTypeStr=boolean
      settings: AttributesFormatString=OFM_OBJ_MOVINGSTATE_E.MOVING = 2
  Compare To Constant7 : simulink/Logic and Bit Operations/Compare To Constant  relop===  const=OFM_OBJ_MOVINGSTATE_E.MOVING_SLOWLY  OutDataTypeStr=boolean
      settings: AttributesFormatString=OFM_OBJ_MOVINGSTATE_E.MOVING_SLOWLY = 5
  Compare To Constant8 : simulink/Logic and Bit Operations/Compare To Constant  relop===  const=OFM_OBJ_MOVINGSTATE_E.UNKNOWN  OutDataTypeStr=boolean
      settings: AttributesFormatString=OFM_OBJ_MOVINGSTATE_E.UNKNOWN = 1
  Compare To Constant9 : simulink/Logic and Bit Operations/Compare To Constant  relop===  const=OFM_OBJ_MOVINGSTATE_E.STATIONARY  OutDataTypeStr=boolean
      settings: AttributesFormatString=OFM_OBJ_MOVINGSTATE_E.STATIONARY = 3
  Constant : Constant  OutDataTypeStr=boolean
  Data Type Conversion1 : DataTypeConversion  OutDataTypeStr=Enum: OFM_OBJ_MOVINGSTATE_E
  Logical Operator15 : Logic  AllPortsSameDT=off  OutDataTypeStr=boolean
  Logical Operator3 : Logic  AllPortsSameDT=off  OutDataTypeStr=boolean
  Logical Operator5 : Logic  Operator=OR  Inputs=4  AllPortsSameDT=off  OutDataTypeStr=boolean
  Logical Operator6 : Logic  Operator=OR  AllPortsSameDT=off  OutDataTypeStr=boolean
  Logical Operator7 : Logic  Operator=OR  Inputs=3  AllPortsSameDT=off  OutDataTypeStr=boolean
  Logical Operator8 : Logic  Operator=OR  AllPortsSameDT=off  OutDataTypeStr=boolean
  Switch : Switch  Criteria=u2 > Threshold
  TOS_HWA_RightFront_FusType : Outport
  wires:
  PP_ObjFusType_FR_Confirm/1 -> Compare To Constant12/1
  Logical Operator5/1 -> Logical Operator15/2
  Compare To Constant6/1 -> Logical Operator5/1
  PP_ObjFusType_FC_Confirm/1 -> Compare To Constant13/1, Compare To Constant11/1
  Compare To Constant8/1 -> Logical Operator7/2
  Compare To Constant12/1 -> Logical Operator8/1
  Compare To Constant11/1 -> Logical Operator8/2
  Compare To Constant10/1 -> Logical Operator5/3
  Data Type Conversion1/1 -> Compare To Constant6/1, Compare To Constant9/1, Compare To Constant8/1, Compare To Constant10/1, Compare To Constant7/1
  Logical Operator15/1 -> Logical Operator6/1
  Logical Operator7/1 -> Logical Operator3/2
  Compare To Constant9/1 -> Logical Operator7/1
  Compare To Constant13/1 -> Logical Operator3/1
  Compare To Constant7/1 -> Logical Operator5/2
  Logical Operator8/1 -> Logical Operator15/1
  object_MovingState/1 -> Data Type Conversion1/1
  Logical Operator3/1 -> Logical Operator6/2
  Logical Operator6/1 -> Switch/1
  HWA_MovState_InternalSig/1 -> Compare To Constant1/1, Compare To Constant3/1
  Compare To Constant3/1 -> Logical Operator5/4
  Compare To Constant1/1 -> Logical Operator7/3
  Object_DX/1 -> Compare To Constant2/1
  Switch/1 -> TOS_HWA_RightFront_FusType/1
  Compare To Constant2/1 -> Switch/2
  Constant/1 -> Switch/3

== system PubIfDecisionTOS_MDL/TOS_20201112/TOS_2012080320/TOS/LC_LCKie_ELK/TOS_HWA/RightLane/TOS_HWA_RightLane/TOS_HWA_RightLane/TOS_HWA/HWA_RightLane/HWA_RightLane_Front/HWA_RightFront_TargMovDir ==
  HWA_MovingDir_InternalSig : Inport
  Compare To Constant3 : simulink/Logic and Bit Operations/Compare To Constant  relop===  const=C_TOS_HWA_MovingDir_Vaild  OutDataTypeStr=boolean
      settings: AttributesFormatString=C_TOS_HWA_MovingDir_Vaild = 1
  TOS_HWA_RightFront_TargMovDir : Outport
  wires:
  HWA_MovingDir_InternalSig/1 -> Compare To Constant3/1
  Compare To Constant3/1 -> TOS_HWA_RightFront_TargMovDir/1

== system PubIfDecisionTOS_MDL/TOS_20201112/TOS_2012080320/TOS/LC_LCKie_ELK/TOS_HWA/RightLane/TOS_HWA_RightLane/TOS_HWA_RightLane/TOS_HWA/HWA_RightLane/HWA_RightLane_Front/HWA_RightRear_Default ==
  Constant{,2..6} (6 alike) : Constant  Value=0  OutDataTypeStr=boolean
  TOS_HWA_RightRear_TargConfirm_b : Outport
  TOS_HWA_RightRear_MovState_ObserVale : Outport  Port=2
  TOS_HWA_RightRear_FusionType_ObserVale : Outport  Port=3
  TOS_HWA_InRightLane_Rear_Flag_ObserVale : Outport  Port=4
  TOS_HWA_RightRear_TargetMovingDir_ObserVale : Outport  Port=5
  TOS_HWA_RightRear_DyConfirm_ObserVale : Outport  Port=6
  wires:
  Constant/1 -> TOS_HWA_RightRear_TargConfirm_b/1
  Constant3/1 -> TOS_HWA_RightRear_FusionType_ObserVale/1
  Constant2/1 -> TOS_HWA_RightRear_MovState_ObserVale/1
  Constant6/1 -> TOS_HWA_RightRear_DyConfirm_ObserVale/1
  Constant5/1 -> TOS_HWA_RightRear_TargetMovingDir_ObserVale/1
  Constant4/1 -> TOS_HWA_InRightLane_Rear_Flag_ObserVale/1

== system PubIfDecisionTOS_MDL/TOS_20201112/TOS_2012080320/TOS/LC_LCKie_ELK/TOS_HWA/RightLane/TOS_HWA_RightLane/TOS_HWA_RightLane/TOS_HWA/HWA_RightLane/HWA_RightLane_Rear/HWA_InRightLane_Flag ==
  TOS_TLJ_RightLaneConfirm_Flag : Inport
  Compare To Constant3 : simulink/Logic and Bit Operations/Compare To Constant  relop===  const=C_TOS_HWA_RightLaneFlag  OutDataTypeStr=boolean
      settings: AttributesFormatString=C_TOS_HWA_RightLaneFlag = 1
  TOS_HWA_InRightLane_Flag : Outport
  wires:
  TOS_TLJ_RightLaneConfirm_Flag/1 -> Compare To Constant3/1
  Compare To Constant3/1 -> TOS_HWA_InRightLane_Flag/1

== system PubIfDecisionTOS_MDL/TOS_20201112/TOS_2012080320/TOS/LC_LCKie_ELK/TOS_HWA/RightLane/TOS_HWA_RightLane/TOS_HWA_RightLane/TOS_HWA/HWA_RightLane/HWA_RightLane_Rear/HWA_RightFront_Default ==
  Constant{1,7..9} (4 alike) : Constant  Value=0  OutDataTypeStr=boolean
  TOS_HWA_RightFront_TargConfirm_b : Outport
  TOS_HWA_RightFront_FusType_ObserVale : Outport  Port=2
  TOS_HWA_InRightLane_Front_Flag_ObserVale : Outport  Port=3
  TOS_HWA_RightFront_TargMovDir_ObserVale : Outport  Port=4
  wires:
  Constant8/1 -> TOS_HWA_InRightLane_Front_Flag_ObserVale/1
  Constant9/1 -> TOS_HWA_RightFront_TargMovDir_ObserVale/1
  Constant7/1 -> TOS_HWA_RightFront_FusType_ObserVale/1
  Constant1/1 -> TOS_HWA_RightFront_TargConfirm_b/1

== system PubIfDecisionTOS_MDL/TOS_20201112/TOS_2012080320/TOS/LC_LCKie_ELK/TOS_HWA/RightLane/TOS_HWA_RightLane/TOS_HWA_RightLane/TOS_HWA/HWA_RightLane/HWA_RightLane_Rear/HWA_RightRear_DyConfirm ==
  Object_DY : Inport
  Object_DX : Inport  Port=2
  Abs1 : Abs
  Abs2 : Abs
  Relational Operator1 : RelationalOperator  Operator=<=  OutDataTypeStr=boolean  RndMeth=Simplest
  data3 : Lookup_n-D  NumberOfTableDimensions=1  BreakpointsForDimension1=[0,20,40,60,80,100,120]  Table=[5.75,5.75,5.75,5.75,5.75,5.75,5.75]  RndMeth=Simplest  InputSameDT=on
  TOS_HWA_RightRear_DyConfirm : Outport
  wires:
  Object_DX/1 -> Abs2/1
  Abs2/1 -> data3/1
  data3/1 -> Relational Operator1/2
  Object_DY/1 -> Abs1/1
  Abs1/1 -> Relational Operator1/1
  Relational Operator1/1 -> TOS_HWA_RightRear_DyConfirm/1

== system PubIfDecisionTOS_MDL/TOS_20201112/TOS_2012080320/TOS/LC_LCKie_ELK/TOS_HWA/RightLane/TOS_HWA_RightLane/TOS_HWA_RightLane/TOS_HWA/HWA_RightLane/HWA_RightLane_Rear/HWA_RightRear_FusionType ==
  Object_FusType : Inport
  Object_DX : Inport  Port=2
  Compare To Constant2 : simulink/Logic and Bit Operations/Compare To Constant  relop=<  const=P_TOS_RefPoint_FixDis_dx1_m  OutDataTypeStr=boolean
      settings: AttributesFormatString=P_TOS_RefPoint_FixDis_dx1_m= -3 m
  Constant : Constant  OutDataTypeStr=boolean
  FusionType : Subsystem
  Switch : Switch  Criteria=u2 > Threshold
  TOS_HWA_RightRear_FusionType : Outport
  wires:
  Object_FusType/1 -> FusionType/1(Object_FusType)
  FusionType/1(TOS_HWA_FusionType) -> Switch/1
  Object_DX/1 -> Compare To Constant2/1
  Compare To Constant2/1 -> Switch/2
  Switch/1 -> TOS_HWA_RightRear_FusionType/1
  Constant/1 -> Switch/3

== system PubIfDecisionTOS_MDL/TOS_20201112/TOS_2012080320/TOS/LC_LCKie_ELK/TOS_HWA/RightLane/TOS_HWA_RightLane/TOS_HWA_RightLane/TOS_HWA/HWA_RightLane/HWA_RightLane_Rear/HWA_RightRear_MovState ==
  HWA_MovState_InternalSig : Inport
  Compare To Constant3 : simulink/Logic and Bit Operations/Compare To Constant  relop===  const=C_TOS_HWA_MovState_Vaild  OutDataTypeStr=boolean
      settings: AttributesFormatString=C_TOS_HWA_MovState_Vaild = 1
  TOS_HWA_RightRear_MovState : Outport
  wires:
  HWA_MovState_InternalSig/1 -> Compare To Constant3/1
  Compare To Constant3/1 -> TOS_HWA_RightRear_MovState/1

== system PubIfDecisionTOS_MDL/TOS_20201112/TOS_2012080320/TOS/LC_LCKie_ELK/TOS_HWA/RightLane/TOS_HWA_RightLane/TOS_HWA_RightLane/TOS_HWA/HWA_RightLane/HWA_RightLane_Rear/HWA_RightRear_TargetMovingDir ==
  HWA_MovingDir_InternalSig : Inport
  Compare To Constant3 : simulink/Logic and Bit Operations/Compare To Constant  relop===  const=C_TOS_HWA_MovingDir_Vaild  OutDataTypeStr=boolean
      settings: AttributesFormatString=C_TOS_HWA_MovingDir_Vaild = 1
  TOS_HWA_RightRear_TargetMovingDir : Outport
  wires:
  HWA_MovingDir_InternalSig/1 -> Compare To Constant3/1
  Compare To Constant3/1 -> TOS_HWA_RightRear_TargetMovingDir/1

== system PubIfDecisionTOS_MDL/TOS_20201112/TOS_2012080320/TOS/ACC/TOS_ACCCurrentLane/ACC_CurrentLane_Target/TOS_ACC_P0/ACC_P0_Targe/ACC_P0_Targe/TOS_ACC_TargetMovingDirConfirm/TOS_ACC_TargetMovingDirConfirm_V2011170316(备份)/TOS_ACCMovingDirAborDly/If Action Subsystem ==
  TOS_ACCMovingDir : Inport
  Action Port : ActionPort
  TOS_ACCMovingDirFilt : Outport
  wires:
  TOS_ACCMovingDir/1 -> TOS_ACCMovingDirFilt/1

== system PubIfDecisionTOS_MDL/TOS_20201112/TOS_2012080320/TOS/ACC/TOS_ACCCurrentLane/ACC_CurrentLane_Target/TOS_ACC_P0/ACC_P0_Targe/ACC_P0_Targe/TOS_ACC_TargetMovingDirConfirm/TOS_ACC_TargetMovingDirConfirm_V2011170316(备份)/TOS_ACCMovingDirAborDly/If Action Subsystem1 ==
  TOS_ACCMovingDir : Inport
  Action Port : ActionPort
  Constant : Constant  Value=0.15
  Constant4 : Constant  Value=0.05
  StateDelayAbortion : TOS_LIB/StateDelayAbortion  SystemSampleTime=-1  VariantActivationTime=update diagram  Latency=0  AutoFrameSizeCalculation=off
  TOS_ACCMovingDirFilt : Outport
  wires:
  StateDelayAbortion/1 -> TOS_ACCMovingDirFilt/1
  Constant/1 -> StateDelayAbortion/2
  Constant4/1 -> StateDelayAbortion/3
  TOS_ACCMovingDir/1 -> StateDelayAbortion/1

== system PubIfDecisionTOS_MDL/TOS_20201112/TOS_2012080320/TOS/ACC/TOS_ACCCurrentLane/ACC_CurrentLane_Target/TOS_ACC_P0/ACC_P0_Targe/ACC_P0_Targe/TOS_ACC_TargetMovingDirConfirm/TOS_ACC_TargetMovingDirConfirm_V2011170316(备份)/TOS_ACCMovingDirAborDly/Subsystem ==
  ACC_TargetP0_ID_K1 : Inport
  ObjectID : Inport  Port=2
  Relational Operator : RelationalOperator  Operator===  OutDataTypeStr=boolean  RndMeth=Simplest
  ACC_SameTargetP0 : Outport
  wires:
  ObjectID/1 -> Relational Operator/2
  Relational Operator/1 -> ACC_SameTargetP0/1
  ACC_TargetP0_ID_K1/1 -> Relational Operator/1

== system PubIfDecisionTOS_MDL/TOS_20201112/TOS_2012080320/TOS/AEB/TOS_AEBLong/AEBLong_Confirm/AEBLong/AEBLong_TrgConfirm/AEBLongTrgJudg/TOS_AEBLong_TargetMovingDir/ObjMovingDirSignalProcessing1/MappingObjInCurveLaneVXVY/ObjectInCurveLaneMappingVXVY ==
  note: 目标到中心线之间距离dyc
  Object_DX : Inport
  Object_VX : Inport  Port=2
  Object_VY : Inport  Port=3
  line01_C1 : Inport  Port=4
  line01_C2 : Inport  Port=5
  line01_dDisStart : Inport  Port=6
  line01_dDisEnd : Inport  Port=7
  line02_C1 : Inport  Port=8
  line02_C2 : Inport  Port=9
  line02_dDisStart : Inport  Port=10
  line02_dDisEnd : Inport  Port=11
  line03_C1 : Inport  Port=12
  line03_C2 : Inport  Port=13
  line03_dDisStart : Inport  Port=14
  line03_dDisEnd : Inport  Port=15
  line04_C1 : Inport  Port=16
  line04_C2 : Inport  Port=17
  line04_dDisStart : Inport  Port=18
  line04_dDisEnd : Inport  Port=19
  line05_C1 : Inport  Port=20
  line05_C2 : Inport  Port=21
  line05_dDisStart : Inport  Port=22
  line05_dDisEnd : Inport  Port=23
  line06_C1 : Inport  Port=24
  line06_C2 : Inport  Port=25
  line06_dDisStart : Inport  Port=26
  line06_dDisEnd : Inport  Port=27
  BaseObjDx_C1_C2_Calculate : Subsystem
  Object_MappingVXVYCalculate : Subsystem
  Object_MappingVX : Outport
  Object_MappingVY : Outport  Port=2
  wires:
  Object_MappingVXVYCalculate/1(Object_MappingVX) -> Object_MappingVX/1
  BaseObjDx_C1_C2_Calculate/1(BaseObjDx_C1_C2) -> Object_MappingVXVYCalculate/3(BaseObjDx_C1_C2)
  Object_VX/1 -> Object_MappingVXVYCalculate/1(Object_VX)
  Object_VY/1 -> Object_MappingVXVYCalculate/2(Object_VY)
  line01_dDisStart/1 -> BaseObjDx_C1_C2_Calculate/4(line01_dDisStart)
  line01_dDisEnd/1 -> BaseObjDx_C1_C2_Calculate/5(line01_dDisEnd)
  line01_C2/1 -> BaseObjDx_C1_C2_Calculate/3(line01_C2)
  line01_C1/1 -> BaseObjDx_C1_C2_Calculate/2(line01_C1)
  line02_C1/1 -> BaseObjDx_C1_C2_Calculate/6(line02_C1)
  line02_C2/1 -> BaseObjDx_C1_C2_Calculate/7(line02_C2)
  line02_dDisStart/1 -> BaseObjDx_C1_C2_Calculate/8(line02_dDisStart)
  Object_DX/1 -> BaseObjDx_C1_C2_Calculate/1(Object_DX)
  line02_dDisEnd/1 -> BaseObjDx_C1_C2_Calculate/9(line02_dDisEnd)
  line03_C1/1 -> BaseObjDx_C1_C2_Calculate/10(line03_C1)
  line03_dDisStart/1 -> BaseObjDx_C1_C2_Calculate/12(line03_dDisStart)
  line03_C2/1 -> BaseObjDx_C1_C2_Calculate/11(line03_C2)
  line03_dDisEnd/1 -> BaseObjDx_C1_C2_Calculate/13(line03_dDisEnd)
  line04_C1/1 -> BaseObjDx_C1_C2_Calculate/14(line04_C1)
  line04_C2/1 -> BaseObjDx_C1_C2_Calculate/15(line04_C2)
  line04_dDisStart/1 -> BaseObjDx_C1_C2_Calculate/16(line04_dDisStart)
  line04_dDisEnd/1 -> BaseObjDx_C1_C2_Calculate/17(line04_dDisEnd)
  line05_C1/1 -> BaseObjDx_C1_C2_Calculate/18(line05_C1)
  line05_C2/1 -> BaseObjDx_C1_C2_Calculate/19(line05_C2)
  line05_dDisStart/1 -> BaseObjDx_C1_C2_Calculate/20(line05_dDisStart)
  line05_dDisEnd/1 -> BaseObjDx_C1_C2_Calculate/21(line05_dDisEnd)
  line06_C1/1 -> BaseObjDx_C1_C2_Calculate/22(line06_C1)
  line06_C2/1 -> BaseObjDx_C1_C2_Calculate/23(line06_C2)
  line06_dDisStart/1 -> BaseObjDx_C1_C2_Calculate/24(line06_dDisStart)
  line06_dDisEnd/1 -> BaseObjDx_C1_C2_Calculate/25(line06_dDisEnd)
  Object_MappingVXVYCalculate/2(Object_MappingVY) -> Object_MappingVY/1

== system PubIfDecisionTOS_MDL/TOS_20201112/TOS_2012080320/TOS/AEB/TOS_AEBLong/AEBLong_Confirm/AEBLong/AEBLong_TrgConfirm/AEBLongTrgJudg/TOS_AEBLong_TargetMovingDir/ObjMovingDirSignalProcessing1/MappingObjInCurveLaneVXVY/ObjectVYVXAngle ==
  Object_MappingVX : Inport
  Object_MappingVY : Inport  Port=2
  Object_VXMeanFilt : Subsystem
  Object_VYMeanFilt : Subsystem
  Object_VYVXAngle : Subsystem
  ObjectVYVXAngle : Outport
  ObjectMappingVY : Outport  Port=2
  ObjectMappingVX : Outport  Port=3
  wires:
  Object_MappingVX/1 -> ObjectMappingVX/1, Object_VXMeanFilt/1(Object_VX)
  Object_VYMeanFilt/1(ObjectVYFilt) -> Object_VYVXAngle/1(ObjectVYFilt)
  Object_VXMeanFilt/1(ObjectVXFilt) -> Object_VYVXAngle/2(ObjectVXFilt)
  Object_VYVXAngle/1(Object_VYVXAngle) -> ObjectVYVXAngle/1
  Object_MappingVY/1 -> ObjectMappingVY/1, Object_VYMeanFilt/1(Object_VY)

== system PubIfDecisionTOS_MDL/TOS_20201112/TOS_2012080320/TOS/AEB/TOS_AEBLong/AEBLong_Confirm/AEBLong/AEBLong_TrgConfirm/AEBLongTrgJudg/TOS_AEBLong_TargetMovingDir/ObjMovingDirSignalProcessing1/Oncoming_MovingDir_StrightLane/OncomingVXCondition ==
  note: VXThre
  Object_MappingVX : Inport
  Object_DX : Inport  Port=2
  Object_DY : Inport  Port=3
  Abs : Abs
  Abs1 : Abs
  Product : Product
  Relational Operator1 : RelationalOperator  Operator=<  OutDataTypeStr=boolean  RndMeth=Nearest
  VXThre_BaseDX : Lookup_n-D  NumberOfTableDimensions=1  BreakpointsForDimension1=[0,30,60,90,120,150]  Table=[0,-1,-2,-2.8,-2.9,-2.9]  InternalRulePriority=Speed  RndMeth=Simplest  InputSameDT=on
  VXThre_BaseDY : Lookup_n-D  NumberOfTableDimensions=1  BreakpointsForDimension1=[0,5,10,15,20,30,50]  Table=[1,1.1,1.12,1.15,1.2,1.2,1.2]  InternalRulePriority=Speed  RndMeth=Simplest  InputSameDT=on
  OncomingVXFlg : Outport
  wires:
  Object_DY/1 -> Abs/1
  VXThre_BaseDY/1 -> Product/2
  Object_DX/1 -> Abs1/1
  Relational Operator1/1 -> OncomingVXFlg/1
  VXThre_BaseDX/1 -> Product/1
  Product/1 -> Relational Operator1/2
  Object_MappingVX/1 -> Relational Operator1/1
  Abs/1 -> VXThre_BaseDY/1
  Abs1/1 -> VXThre_BaseDX/1
